simulink model "gmsk_softdecision"  (Simulink 6.0)
settings: Solver=VariableStepDiscrete  SolverMode=SingleTasking  StartTime=0.0  StopTime=1e3  RelTol=1e-3
undefined symbols (not defined in the file or in its folder): Fs, Low, slcm
libraries: dspsigops x8, commsink2 x4, commcnvcod2 x3, simulink x3, commsrccod2 x2, commutil2 x2, dspsrcs4 x2, commsequence2 x2, dspbuff3 x2, commchan2 x1, commrandsrc2 x1, dspsnks4 x1
CloseFcn:
  | clear gmskSigsOut;
settings Model: Creator=arodrigu  LastModifiedBy=arodrigu  ExtModeAutoUpdateStatusClock=off  ProdHWDeviceType=Specified
settings DataIOCC: SaveOutput=off  SaveTime=off  SignalLoggingName=gmskSigsOut
settings OptimizationCC: BooleanDataType=off
settings DebuggingCC: CheckExecutionContextPreStartOutputMsg=on  CheckExecutionContextRuntimeOutputMsg=on  SolverPrmCheckMsg=none  InheritedTsInSrcMsg=none
settings HardwareCC: ProdHWDeviceType=Specified
settings ModelReferenceCC: UpdateModelReferenceTargets=IfOutOfDate

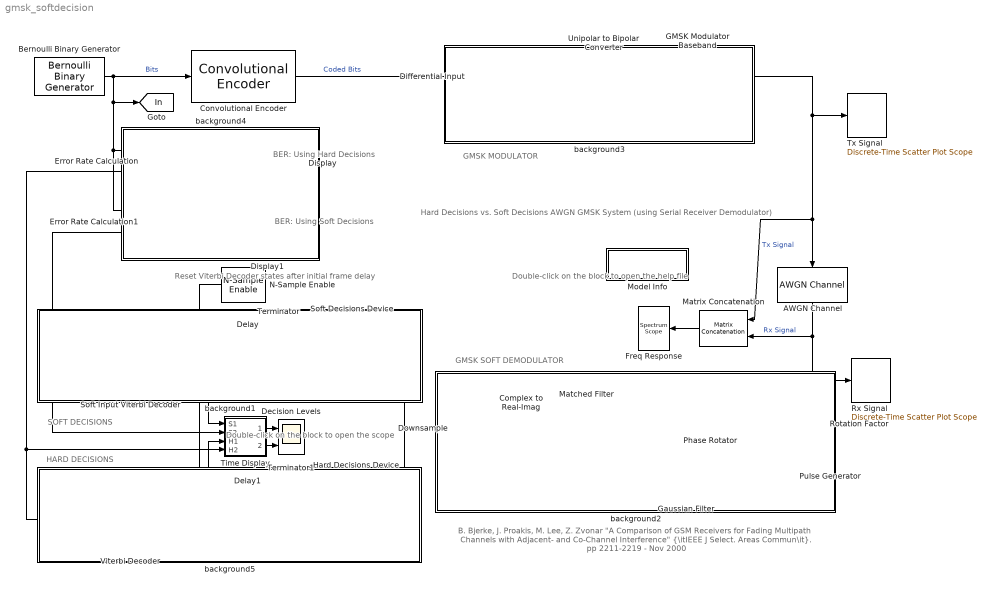
== system gmsk_softdecision ==
  note: BER:
      | Using Hard Decisions
  note: Hard Decisions vs. Soft Decisions
      | AWGN GMSK System
      | (using Serial Receiver Demodulator)
  note: BER:
      | Using Soft Decisions
  note: SOFT DECISIONS
  note: HARD DECISIONS
  note: GMSK SOFT DEMODULATOR
  note: B. Bjerke, J. Proakis, M. Lee, Z. Zvonar
      |  "A Comparison of GSM Receivers for Fading Multipath Channels
      | with Adjacent- and Co-Channel Interference"
      | {\itIEEE J Select. Areas Commun\it}. pp 2211-2219 - Nov 2000
  note: Reset Viterbi Decoder states after
      | initial frame delay
  note: Double-click on the block
      | to open the help file
  note: GMSK MODULATOR
  note: Double-click on
      | the block
      | to open the scope
  AWGN Channel : commchan2/AWGN Channel  Orientation=down  seed=67  noiseMode="Signal to noise ratio  (Es/No)"  EbNodB=10  EsNodB=16  SNRdB=10  bitsPerSym=1  Ps=1  Tsym=1  variance=1
  Bernoulli Binary Generator : commrandsrc2/Bernoulli Binary Generator  P=0.5  seed=61  Ts=1/5  frameBased=on  sampPerFrame=5  orient=off
  Complex to Real-Imag : ComplexToRealImag  Orientation=left  Output=Real
  Convolutional Encoder : commcnvcod2/Convolutional Encoder  trellis=poly2trellis(7, [171 133])  reset=None
  Decision Levels : Scope  NumInputPorts=2
      settings: TimeRange=35  YMin=0~0  YMax=8~1.2
  Delay : dspsigops/Delay  Orientation=left  dly_unit=Samples  delay=5  ic_detail=off  dif_ic_for_ch=off  dif_ic_for_dly=off  ic=0  reset_popup=None
  Delay1 : dspsigops/Delay  Orientation=left  dly_unit=Samples  delay=5  ic_detail=off  dif_ic_for_ch=off  dif_ic_for_dly=off  ic=0  reset_popup=None
  Differential Input : Subsystem  PropExecContextAcrossSSBoundary=on
  Display : Display
  Display1 : Display
  Downsample : dspsigops/Downsample  Orientation=left  N=8  phase=0  ic=0  smode=Allow multirate  fmode=Maintain input frame rate
  Error Rate Calculation : commsink2/Error Rate Calculation  N=34+5  st_delay=0  cp_mode=Entire frame  subframe=[]  PMode=Port  WsName=ErrorVec  RsMode2=off  stop=off  numErr=1e2  maxBits=1e4
  Error Rate Calculation1 : commsink2/Error Rate Calculation  N=34+5  st_delay=0  cp_mode=Entire frame  subframe=[]  PMode=Port  WsName=ErrorVec  RsMode2=off  stop=off  numErr=100  maxBits=1e6
  Freq Response : dspsnks4/Spectrum Scope  Orientation=left  ScopeProperties=on  Domain=Frequency  HorizSpan=1  UseBuffer=on  BufferSize=128*4  Overlap=48  inpFftLenInherit=off  FFTlength=128  numAvg=10  DisplayProperties=off  AxisGrid=on  Memory=off  FrameNumber=off  AxisLegend=on  AxisZoom=off  OpenScopeAtSimStart=on  OpenScopeImmediately=off  FigPos=[229 398 381 306]  AxisProperties=off  XUnits=Hertz  XRange=[-Fs/2...Fs/2]  InheritXIncr=on  XIncr=1.0  XLabel=Samples  YUnits=dB  YLabel=Magnitude, dB  LineProperties=off  LineColors=[0 0 0]|[1 0 0]
      settings: YMin=-123.326456268335  YMax=23.4309325701245
  GMSK Modulator Baseband : commdigbbndcpm2/GMSK Modulator Baseband  inputType=Integer  BT=.3  pulseLength=4  preHistory=1  phaseOffset=0  samplesPerSymbol=8
  Gaussian Filter : commfilt2/Gaussian Filter  Orientation=left  N=8  BT=0.3  D=2  sampMode=Frame-based  normMode=Sum of coefficients  filterGain=1  checkCoeff=off  variableName=gaussFilt2  launchFVT=off
  Hard Decisions Device : commsrccod2/Quantizing Encoder  Orientation=left  partition=0  codebook=[1 0]
  Matched Filter : dsparch4/Digital Filter  Orientation=left  DialogController=dspDDGCreate  DialogControllerArgs=DataTag0  TypePopup=FIR (all zeros)  IIRFiltStruct=Direct form II transposed  AllPoleFiltStruct=Direct form  FIRFiltStruct=Direct form  CoeffSource=Input port(s)  NumCoeffs=[1 2]  DenCoeffs=[1 0.1]  BiQuadCoeffs=[1 0.3 0.4 1 0.1 0.2]  LatticeCoeffs=[0.2 0.4]  denIgnore=on  FiltPerSampPopup=One filter per frame  IC=0  ICnum=0  ICden=0  roundingMode=Floor  overflowMode=off  ScaleValues=1  scaleValueFracLength=14  stageInFracLength=15  stageOutFracLength=15
  Matrix Concatenation : simulink/Math Operations/Matrix Concatenation  Orientation=left  numInports=2  catMethod=Horizontal
  Model Info : Subsystem  LoadFcn=slcm LoadBlock;  InitFcn=slcm('UpdateAllCMBlocksInThisModelInit')  PropExecContextAcrossSSBoundary=on  mask(CMBlock){InitialSaveTempField=, InitialBlockCM=None, BlockCM=None, Frame=on, SaveTempField=, DisplayStringWithTags=Info, MaskDisplayString=Info, HorizontalTextAlignment=Center, LeftAlignmentValue=0.5, SourceBlockDiagram=gmsk_softdecision, TagMaxNumber=20, CMTag1=, CMTag2=, CMTag3=, CMTag4=, CMTag5=, CMTag6=, CMTag7=, CMTag8=, CMTag9=, CMTag10=, CMTag11=, CMTag12=, CMTag13=, CMTag14=, CMTag15=, CMTag16=, CMTag17=, CMTag18=, CMTag19=, CMTag20=}
      mask help: This block allows revision control information to be displayed within the model.
      settings: CopyFcn=slcm CopyBlock;  DeleteFcn=slcm Cancel;  PostSaveFcn=slcm('UpdateAllCMBlocksInThisModel')  NameChangeFcn=slcm Rename;  OpenFcn=commdemohelp;
      mask Display: text(str2num(LeftAlignmentValue), 0.5, MaskDisplayString, 'HorizontalAlignment', HorizontalTextAlignment)
  N-Sample Enable : dspswit3/N-Sample Enable  Orientation=left  N=1  ActiveLevel=Low (0)  reset=off  TriggerType=Rising edge  Ts=1  DataType=Logical
  Phase Rotator : commutil2/Complex Phase Shift  Orientation=left
  Pulse Generator : Subsystem  Orientation=left  PropExecContextAcrossSSBoundary=on
      mask Display: plot(0,0,45,100,[5 10 10 10 40],[0 0 60 0 0]+20)
  Rotation Factor : Subsystem  Orientation=left  PropExecContextAcrossSSBoundary=on
  Rx Signal : commsink2/Discrete-Time Scatter Plot Scope  Tag=ScatterPlot  sampPerSymb=8  offsetEye=0  numTraces=400  numNewFrames=10  LineMarkers=.  LineColors=b  fading=on  render=on  AxisGrid=on  xMin=-3.7226102881776  xMax=3.4540054001378  yMin=-3.48544462250425  yMax=3.69117106581115  inphaseLabel=.  quadratureLabel=.  openScopeAtSimStart=on  FrameNumber=off  FigPos=[619 138 268 268]  figTitle=.  numLinesMax=8  block_type_=scatter
  Soft Decisions Device : commsrccod2/Quantizing Encoder  Orientation=left  partition=[-.75 -.5 -.25 0 .25 .5 .75]  codebook=[7 6 5 4 3 2 1 0]
  Soft Input Viterbi Decoder : commcnvcod2/Viterbi Decoder  Orientation=left  trellis=poly2trellis(7, [171 133])  dectype=Soft Decision  nsdecb=3  tbdepth=34  opmode=Continuous  reset=on
  Terminator : Terminator
  Terminator1 : Terminator
  Time Display : Subsystem  PropExecContextAcrossSSBoundary=on
  Tx Signal : commsink2/Discrete-Time Scatter Plot Scope  Tag=ScatterPlot  sampPerSymb=8  offsetEye=0  numTraces=400  numNewFrames=10  LineMarkers=.  LineColors=b  fading=on  render=on  AxisGrid=on  xMin=-1.1  xMax=1.105  yMin=-1.1  yMax=1.105  inphaseLabel=.  quadratureLabel=.  openScopeAtSimStart=on  FrameNumber=off  FigPos=[618 456 268 268]  figTitle=.  numLinesMax=8  block_type_=scatter
  Unipolar to Bipolar Converter : commutil2/Unipolar to Bipolar Converter  M=2  polarity=Negative
  Viterbi Decoder : commcnvcod2/Viterbi Decoder  Orientation=left  trellis=poly2trellis(7, [171 133])  dectype=Hard Decision  nsdecb=4  tbdepth=34  opmode=Continuous  reset=on
  background1 : Subsystem  Orientation=left  PropExecContextAcrossSSBoundary=on
      mask Display: disp('')
  background2 : Subsystem  Orientation=left  PropExecContextAcrossSSBoundary=on
      mask Display: disp('')
  background3 : Subsystem  Orientation=left  PropExecContextAcrossSSBoundary=on
      mask Display: disp('')
  background4 : Subsystem  Orientation=left  PropExecContextAcrossSSBoundary=on
      mask Display: disp('')
  background5 : Subsystem  Orientation=left  PropExecContextAcrossSSBoundary=on
      mask Display: disp('')
  tag scope: In=global
  wires:
  Bernoulli Binary Generator/1 -> Convolutional Encoder/1, Error Rate Calculation1/1, Error Rate Calculation/1, [In]  "Bits"
  Differential Input/1(Out1) -> Unipolar to Bipolar Converter/1
  Unipolar to Bipolar Converter/1 -> GMSK Modulator Baseband/1
  Error Rate Calculation/1 -> Display/1
  GMSK Modulator Baseband/1 -> AWGN Channel/1, Matrix Concatenation/1, Tx Signal/1  "Tx Signal"
  Rotation Factor/1(Ph) -> Phase Rotator/2
  Phase Rotator/1 -> Matched Filter/1
  Gaussian Filter/1 -> Matched Filter/2
  Downsample/1 -> Soft Decisions Device/1, Hard Decisions Device/1
  Hard Decisions Device/2 -> Delay1/1
  Convolutional Encoder/1 -> Differential Input/1(In1)  "Coded Bits"
  Viterbi Decoder/1 -> Error Rate Calculation/2, Time Display/4(H2)
  Delay1/1 -> Viterbi Decoder/1, Time Display/3(H1)
  Error Rate Calculation1/1 -> Display1/1
  Soft Input Viterbi Decoder/1 -> Error Rate Calculation1/2, Time Display/2(S2)
  Soft Decisions Device/2 -> Delay/1
  Delay/1 -> Soft Input Viterbi Decoder/1, Time Display/1(S1)
  N-Sample Enable/1 -> Viterbi Decoder/2, Soft Input Viterbi Decoder/2
  Soft Decisions Device/1 -> Terminator/1
  Hard Decisions Device/1 -> Terminator1/1
  Complex to Real-Imag/1 -> Downsample/1
  Pulse Generator/1(Out1) -> Gaussian Filter/1
  Matched Filter/1 -> Complex to Real-Imag/1
  AWGN Channel/1 -> Matrix Concatenation/2, Phase Rotator/1, Rx Signal/1  "Rx Signal"
  Time Display/2(Out2) -> Decision Levels/2
  Time Display/1(Out1) -> Decision Levels/1
  Matrix Concatenation/1 -> Freq Response/1

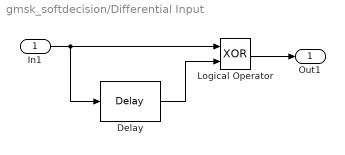
== system gmsk_softdecision/Differential Input ==
  In1 : Inport  LatchInput=off
  Delay : dspsigops/Delay  dly_unit=Samples  delay=1  ic_detail=on  dif_ic_for_ch=off  dif_ic_for_dly=off  ic=0  reset_popup=None
  Logical Operator : Logic  Operator=XOR  AllPortsSameDT=off
  Out1 : Outport
  wires:
  Logical Operator/1 -> Out1/1
  Delay/1 -> Logical Operator/2
  In1/1 -> Delay/1, Logical Operator/1

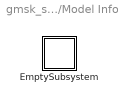
== system gmsk_softdecision/Model Info ==
  EmptySubsystem : Subsystem  PropExecContextAcrossSSBoundary=on

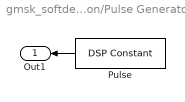
== system gmsk_softdecision/Pulse Generator ==
  Pulse : dspsrcs4/DSP Constant  Orientation=left  Value=[1; zeros(32,1)]  SampleMode=Discrete  discreteOutput=Frame-based  continuousOutput=Sample-based  sampTime=1  framePeriod=1  dataType=Inherit from 'Constant value'  isSigned=on  wordLen=16  udDataType=sfix(16)  fracBitsMode=Best precision  numFracBits=15  InterpretAs1D=-inf  Ts=-inf  FramebasedOutput=-inf
  Out1 : Outport  Orientation=left
  wires:
  Pulse/1 -> Out1/1

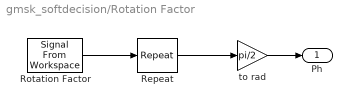
== system gmsk_softdecision/Rotation Factor ==
  Repeat : dspsigops/Repeat  N=8  ic=0  mode=Maintain input frame rate
  Rotation Factor : dspsrcs4/Signal From Workspace  X=[4:-1:1]  Ts=1/10  nsamps=10  OutputAfterFinalValue=Cyclic repetition
  to rad : Gain  Gain=pi/2  SaturateOnIntegerOverflow=on
  Ph : Outport
  wires:
  Rotation Factor/1 -> Repeat/1
  to rad/1 -> Ph/1
  Repeat/1 -> to rad/1

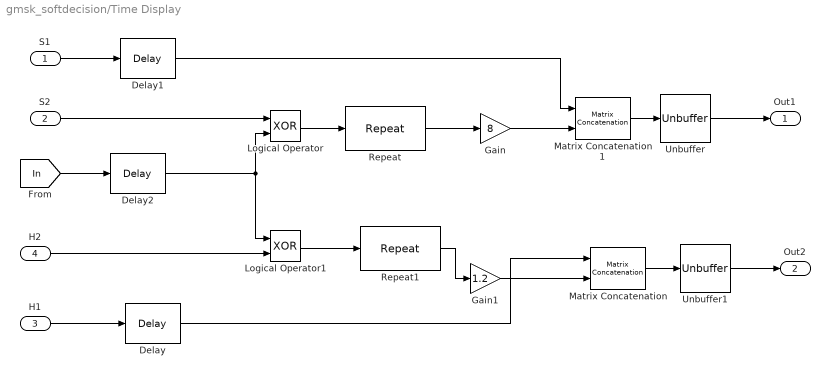
== system gmsk_softdecision/Time Display ==
  S1 : Inport  LatchInput=off
  S2 : Inport  Port=2  LatchInput=off
  H1 : Inport  Port=3  LatchInput=off
  H2 : Inport  Port=4  LatchInput=off
  Delay : dspsigops/Delay  dly_unit=Samples  delay=34  ic_detail=off  dif_ic_for_ch=off  dif_ic_for_dly=off  ic=0  reset_popup=None
  Delay1 : dspsigops/Delay  dly_unit=Samples  delay=34  ic_detail=off  dif_ic_for_ch=off  dif_ic_for_dly=off  ic=0  reset_popup=None
  Delay2 : dspsigops/Delay  dly_unit=Samples  delay=34+5  ic_detail=off  dif_ic_for_ch=off  dif_ic_for_dly=off  ic=0  reset_popup=None
  Gain : Gain  Gain=8
  Gain1 : Gain  Gain=1.2
  Logical Operator : Logic  Operator=XOR  AllPortsSameDT=off
  Logical Operator1 : Logic  Operator=XOR  AllPortsSameDT=off
  Matrix Concatenation : simulink/Math Operations/Matrix Concatenation  numInports=2  catMethod=Horizontal
  Matrix Concatenation1 : simulink/Math Operations/Matrix Concatenation  numInports=2  catMethod=Horizontal
  Repeat : commsequence2/Repeat  N=2  ic=0  mode=Maintain input frame rate
  Repeat1 : commsequence2/Repeat  N=2  ic=0  mode=Maintain input frame rate
  Unbuffer : dspbuff3/Unbuffer  ic=0
  Unbuffer1 : dspbuff3/Unbuffer  ic=0
  Out1 : Outport
  Out2 : Outport  Port=2
  wires:
  S1/1 -> Delay1/1
  S2/1 -> Logical Operator/1
  H2/1 -> Logical Operator1/2
  H1/1 -> Delay/1
  [In] -> Delay2/1
  Delay2/1 -> Logical Operator/2, Logical Operator1/1
  Logical Operator/1 -> Repeat/1
  Logical Operator1/1 -> Repeat1/1
  Delay1/1 -> Matrix Concatenation1/1
  Delay/1 -> Matrix Concatenation/1
  Repeat1/1 -> Gain1/1
  Repeat/1 -> Gain/1
  Matrix Concatenation1/1 -> Unbuffer/1
  Matrix Concatenation/1 -> Unbuffer1/1
  Unbuffer1/1 -> Out2/1
  Unbuffer/1 -> Out1/1
  Gain/1 -> Matrix Concatenation1/2
  Gain1/1 -> Matrix Concatenation/2

== system gmsk_softdecision/background1 ==

== system gmsk_softdecision/background2 ==

== system gmsk_softdecision/background3 ==

== system gmsk_softdecision/background4 ==

== system gmsk_softdecision/background5 ==

== system gmsk_softdecision/Model Info/EmptySubsystem ==
